simulink model "imu"  (R2015b)
settings: Solver=ode5  StartTime=0.0  StopTime=inf  FixedStep=0.02  RelTol=1e-3
libraries: realtime_pacer_lib x1, robotlib x1
settings Model: Creator=root  LastModifiedBy=root

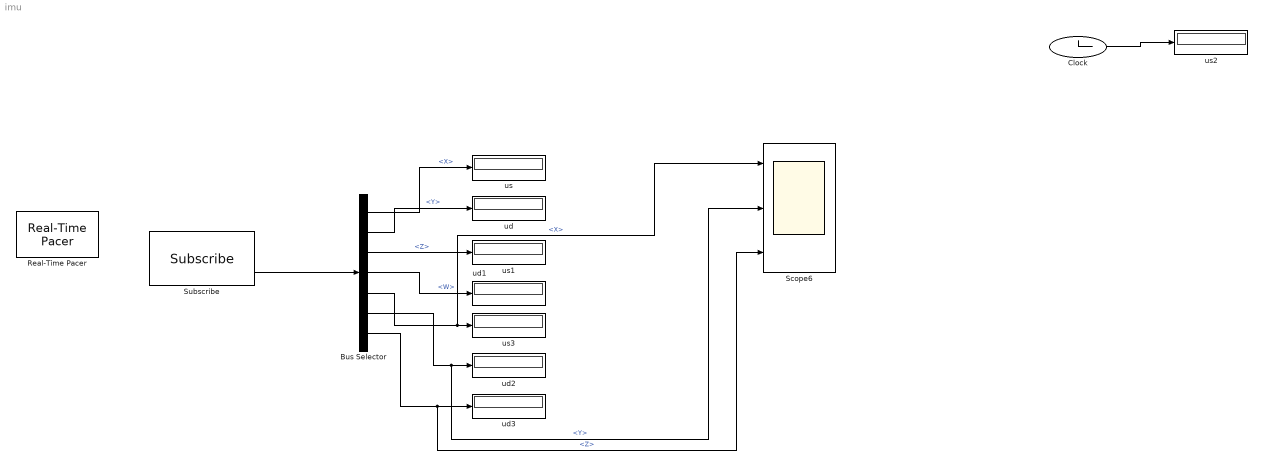
== system imu ==
  Bus Selector : BusSelector  OutputSignals=Orientation.X,Orientation.Y,Orientation.Z,Orientation.W,AngularVelocity.X,AngularVelocity.Y,AngularVelocity.Z
  Clock : Clock
  Real-Time Pacer : realtime_pacer_lib/Real-Time Pacer  simTimePerRealTime=inf
  Scope6 : Scope  NumInputPorts=3
  Subscribe : robotlib/Subscribe  SourceLibraryInfo=This block requires Robotics System Toolbox  topicSource=Select from ROS network  topic=/imu  messageType=sensor_msgs/Imu  sampleTime=-1  messageQueueLength=1
  ud{,1..3} (4 alike) : Display
  us{,1..3} (4 alike) : Display
  wires:
  Subscribe/2 -> Bus Selector/1
  Clock/1 -> us2/1
  Bus Selector/1 -> us/1  "<X>"
  Bus Selector/2 -> ud/1  "<Y>"
  Bus Selector/3 -> us1/1  "<Z>"
  Bus Selector/4 -> ud1/1  "<W>"
  Bus Selector/5 -> Scope6/1, us3/1  "<X>"
  Bus Selector/6 -> Scope6/2, ud2/1  "<Y>"
  Bus Selector/7 -> Scope6/3, ud3/1  "<Z>"
